simulink library "INT_EngBrk_VNTP"  (R2016b)
settings: Solver=VariableStepAuto  StartTime=0.0  StopTime=10.0  RelTol=1e-3
settings Model: Creator=lenovo  LastModifiedBy=lenovo

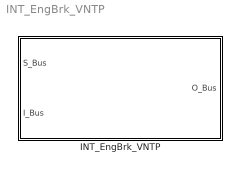
== system INT_EngBrk_VNTP ==
  INT_EngBrk_VNTP : Subsystem

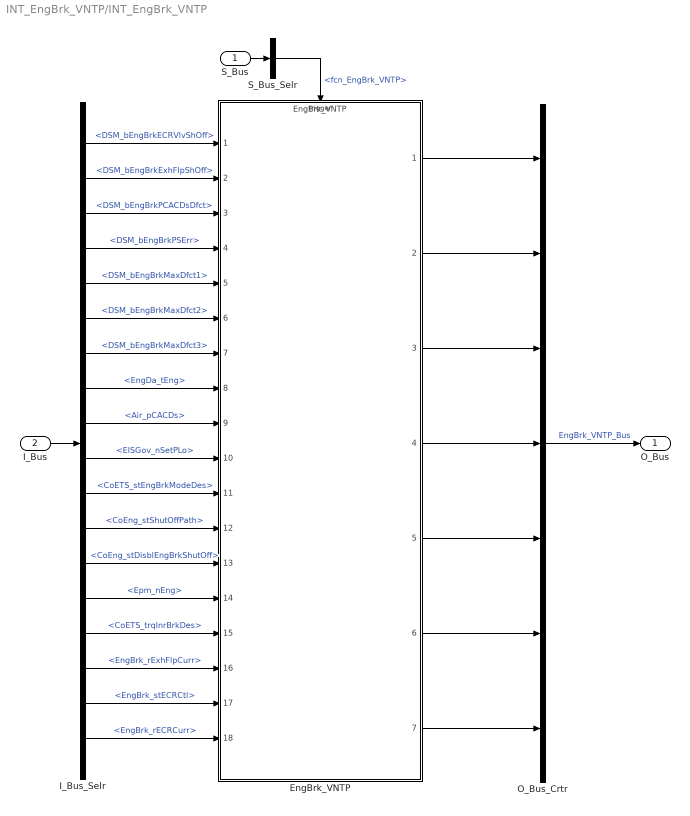
== system INT_EngBrk_VNTP/INT_EngBrk_VNTP ==
  S_Bus : Inport
  I_Bus : Inport  Port=2
  EngBrk_VNTP : ModelReference  ModelNameDialog=EngBrk_VNTP  ModelReferenceVersion=1.9  TriggerPortName=function  TriggerPortTriggerType=function-call  TriggerPortStatesWhenEnabling=held
  I_Bus_Selr : BusSelector  OutputSignals=DSM_bEngBrkECRVlvShOff,DSM_bEngBrkExhFlpShOff,DSM_bEngBrkPCACDsDfct,DSM_bEngBrkPSErr,DSM_bEngBrkMaxDfct1,DSM_bEngBrkMaxDfct2,DSM_bEngBrkMaxDfct3,EngDa_tEng,Air_pCACDs,EISGov_nSetPLo,CoETS_stEngBrkModeDes,CoEng_stShutOffPath,CoEng_stDisblEngBrkShutOff,Epm_nEng,CoETS_trqInrBrkDes,EngBrk_rExhFlpCurr,EngBrk_stECRCtl,EngBrk_rECRCurr
  O_Bus_Crtr : BusCreator  Inputs=7
  S_Bus_Selr : BusSelector  OutputSignals=fcn_EngBrk_VNTP
  O_Bus : Outport
  wires:
  S_Bus_Selr/1 -> EngBrk_VNTP/Trigger  "<fcn_EngBrk_VNTP>"
  S_Bus/1 -> S_Bus_Selr/1
  I_Bus/1 -> I_Bus_Selr/1
  I_Bus_Selr/1 -> EngBrk_VNTP/1  "<DSM_bEngBrkECRVlvShOff>"
  I_Bus_Selr/2 -> EngBrk_VNTP/2  "<DSM_bEngBrkExhFlpShOff>"
  I_Bus_Selr/3 -> EngBrk_VNTP/3  "<DSM_bEngBrkPCACDsDfct>"
  I_Bus_Selr/4 -> EngBrk_VNTP/4  "<DSM_bEngBrkPSErr>"
  I_Bus_Selr/5 -> EngBrk_VNTP/5  "<DSM_bEngBrkMaxDfct1>"
  I_Bus_Selr/6 -> EngBrk_VNTP/6  "<DSM_bEngBrkMaxDfct2>"
  I_Bus_Selr/7 -> EngBrk_VNTP/7  "<DSM_bEngBrkMaxDfct3>"
  I_Bus_Selr/8 -> EngBrk_VNTP/8  "<EngDa_tEng>"
  I_Bus_Selr/9 -> EngBrk_VNTP/9  "<Air_pCACDs>"
  I_Bus_Selr/10 -> EngBrk_VNTP/10  "<EISGov_nSetPLo>"
  I_Bus_Selr/11 -> EngBrk_VNTP/11  "<CoETS_stEngBrkModeDes>"
  I_Bus_Selr/12 -> EngBrk_VNTP/12  "<CoEng_stShutOffPath>"
  I_Bus_Selr/13 -> EngBrk_VNTP/13  "<CoEng_stDisblEngBrkShutOff>"
  I_Bus_Selr/14 -> EngBrk_VNTP/14  "<Epm_nEng>"
  I_Bus_Selr/15 -> EngBrk_VNTP/15  "<CoETS_trqInrBrkDes>"
  I_Bus_Selr/16 -> EngBrk_VNTP/16  "<EngBrk_rExhFlpCurr>"
  I_Bus_Selr/17 -> EngBrk_VNTP/17  "<EngBrk_stECRCtl>"
  I_Bus_Selr/18 -> EngBrk_VNTP/18  "<EngBrk_rECRCurr>"
  O_Bus_Crtr/1 -> O_Bus/1  "EngBrk_VNTP_Bus"
  EngBrk_VNTP/1 -> O_Bus_Crtr/1
  EngBrk_VNTP/2 -> O_Bus_Crtr/2
  EngBrk_VNTP/3 -> O_Bus_Crtr/3
  EngBrk_VNTP/4 -> O_Bus_Crtr/4
  EngBrk_VNTP/5 -> O_Bus_Crtr/5
  EngBrk_VNTP/6 -> O_Bus_Crtr/6
  EngBrk_VNTP/7 -> O_Bus_Crtr/7
